simulink model "s4"  (R2023b)
settings: Solver=ode45  StartTime=0  StopTime=0.3  RelTol=1e-3
settings Model: Creator=t3  LastModifiedBy=t3

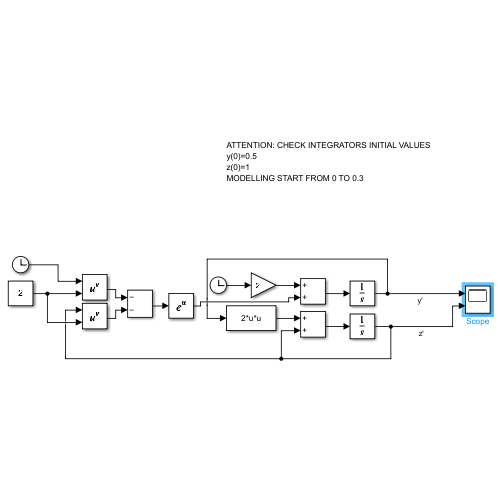
[thumbnail: Simulink's stored preview of the top-level diagram]
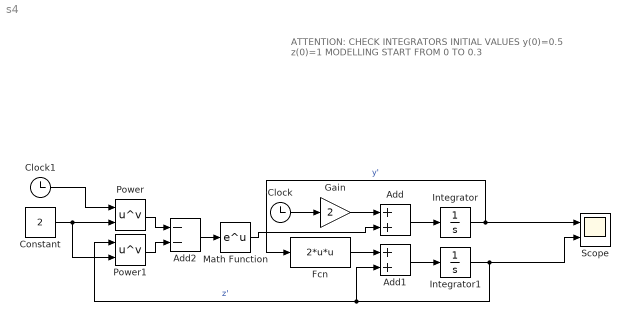
== system s4 ==
  note: ATTENTION: CHECK INTEGRATORS INITIAL VALUES
      | y(0)=0.5
      | z(0)=1
      | MODELLING START FROM 0 TO 0.3
  Add : Sum
  Add1 : Sum
  Add2 : Sum  Inputs=--
  Clock : Clock
  Clock1 : Clock
  Constant : Constant  Value=2
  Fcn : Fcn  Expr=2*u*u
  Gain : Gain  Gain=2
  Integrator : Integrator  InitialCondition=0.5
  Integrator1 : Integrator  InitialCondition=1
  Math Function : Math
  Power : Math  Operator=pow
  Power1 : Math  Operator=pow
  Scope : Scope  NumInputPorts=2
  wires:
  Integrator/1 -> Fcn/1, Scope/1  "y'"
  Integrator1/1 -> Power1/1, Add1/2, Scope/2  "z'"
  Add/1 -> Integrator/1
  Add1/1 -> Integrator1/1
  Fcn/1 -> Add1/1
  Clock/1 -> Gain/1
  Gain/1 -> Add/1
  Power/1 -> Add2/1
  Add2/1 -> Math Function/1
  Math Function/1 -> Add/2
  Constant/1 -> Power/2, Power1/2
  Clock1/1 -> Power/1
  Power1/1 -> Add2/2
